simulink model "five_bots_Observer_Obstacle_1_sin_cir"  (R2019b)
settings: Solver=ode5  StartTime=0.0  StopTime=35.0  FixedStep=0.005  RelTol=1e-3
(part 1 of 3)
settings Model: Creator=a1752760  LastModifiedBy=a1752760
settings DataIOCC: ReturnWorkspaceOutputs=off
settings DebuggingCC: ArithmeticOperatorsInVariantConditions=warning
settings SFSimCC: CustomCodeUndefinedFunction=UseInterfaceOnly

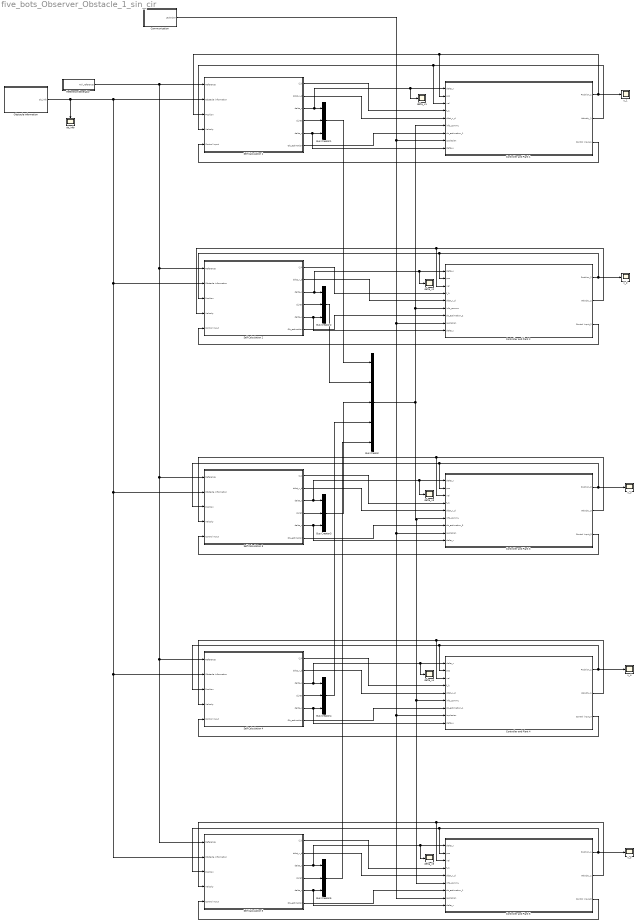
== system five_bots_Observer_Obstacle_1_sin_cir ==
  Bus Creator : BusCreator  Inputs=5
  Bus Creator{1..5} (5 alike) : BusCreator  Inputs=3
  Communication : Subsystem
  Controller and Plant 1 : Subsystem
  Controller and Plant 2 : Subsystem
  Controller and Plant 3 : Subsystem
  Controller and Plant 4 : Subsystem
  Controller and Plant 5 : Subsystem
  Obstacle Information : MATLAB Function  TreatAsAtomicUnit=on
  Reference Generator : Subsystem
  Self Calculation 1 : Subsystem
  Self Calculation 2 : Subsystem
  Self Calculation 3 : Subsystem
  Self Calculation 4 : Subsystem
  Self Calculation 5 : Subsystem
  delta_x{1..5} (5 alike) : Scope
  ob_info : Scope
  x_{1..5} (5 alike) : Scope
  wires:
  Obstacle Information/1(ob_info) -> Self Calculation 5/2(Obstacle information), Self Calculation 4/2(Obstacle information), Self Calculation 3/2(Obstacle information), Self Calculation 2/2(Obstacle information), Self Calculation 1/2(Obstacle information), ob_info/1
  Reference Generator/1(Full_reference) -> Self Calculation 5/1(Reference), Self Calculation 4/1(Reference), Self Calculation 3/1(Reference), Self Calculation 2/1(Reference), Self Calculation 1/1(Reference)
  Controller and Plant 1/1(Position_1) -> Controller and Plant 1/2(pos), Self Calculation 1/3(Position), x_1/1
  Controller and Plant 1/2(Velocity_1) -> Controller and Plant 1/3(vel), Self Calculation 1/4(Velocity)
  Self Calculation 1/1(f_ik) -> Controller and Plant 1/4(f_ik)
  Self Calculation 1/2(ddot_x_d) -> Controller and Plant 1/5(ddot_x_d)
  Self Calculation 1/6(Ob_estimation) -> Controller and Plant 1/7(ob_estimation_1)
  Self Calculation 1/5(delta_v) -> Controller and Plant 1/9(delta_v), Bus Creator1/3
  Self Calculation 1/4(d_hat) -> Bus Creator1/2
  Self Calculation 1/3(delta_x) -> delta_x1/1, Controller and Plant 1/1(delta_x), Bus Creator1/1
  Controller and Plant 1/3(Control input_1) -> Self Calculation 1/5(Control Input)
  Bus Creator1/1 -> Bus Creator/1
  Bus Creator/1 -> Controller and Plant 2/6(info_commu), Controller and Plant 1/6(info_commu), Controller and Plant 5/6(info_commu), Controller and Plant 4/6(info_commu), Controller and Plant 3/6(info_commu)
  Self Calculation 2/1(f_ik) -> Controller and Plant 2/4(f_ik)
  Self Calculation 2/3(delta_x) -> delta_x2/1, Controller and Plant 2/1(delta_x), Bus Creator2/1
  Self Calculation 2/6(Ob_estimation) -> Controller and Plant 2/7(ob_estimation_2)
  Controller and Plant 2/1(Position_2) -> Self Calculation 2/3(Position), Controller and Plant 2/2(pos), x_2/1
  Self Calculation 2/5(delta_v) -> Controller and Plant 2/9(delta_v), Bus Creator2/3
  Controller and Plant 2/2(Velocity_2) -> Controller and Plant 2/3(vel), Self Calculation 2/4(Velocity)
  Self Calculation 2/4(d_hat) -> Bus Creator2/2
  Self Calculation 2/2(ddot_x_d) -> Controller and Plant 2/5(ddot_x_d)
  Controller and Plant 2/3(Control input_2) -> Self Calculation 2/5(Control Input)
  Controller and Plant 3/3(Control input_3) -> Self Calculation 3/5(Control Input)
  Controller and Plant 3/2(Velocity_3) -> Self Calculation 3/4(Velocity), Controller and Plant 3/3(vel)
  Self Calculation 3/1(f_ik) -> Controller and Plant 3/4(f_ik)
  Self Calculation 3/3(delta_x) -> delta_x3/1, Controller and Plant 3/1(delta_x), Bus Creator3/1
  Controller and Plant 3/1(Position_3) -> Self Calculation 3/3(Position), Controller and Plant 3/2(pos), x_3/1
  Self Calculation 3/4(d_hat) -> Bus Creator3/2
  Self Calculation 3/5(delta_v) -> Controller and Plant 3/9(delta_v), Bus Creator3/3
  Self Calculation 3/6(Ob_estimation) -> Controller and Plant 3/7(ob_estimation_3)
  Self Calculation 3/2(ddot_x_d) -> Controller and Plant 3/5(ddot_x_d)
  Controller and Plant 4/3(Control input_4) -> Self Calculation 4/5(Control Input)
  Controller and Plant 4/2(Velocity_1) -> Self Calculation 4/4(Velocity), Controller and Plant 4/3(vel)
  Self Calculation 4/1(f_ik) -> Controller and Plant 4/4(f_ik)
  Self Calculation 4/3(delta_x) -> delta_x4/1, Controller and Plant 4/1(delta_x), Bus Creator4/1
  Controller and Plant 4/1(Position_1) -> Self Calculation 4/3(Position), Controller and Plant 4/2(pos), x_4/1
  Self Calculation 4/4(d_hat) -> Bus Creator4/2
  Self Calculation 4/5(delta_v) -> Controller and Plant 4/9(delta_v), Bus Creator4/3
  Self Calculation 4/6(Ob_estimation) -> Controller and Plant 4/7(ob_estimation_1)
  Self Calculation 4/2(ddot_x_d) -> Controller and Plant 4/5(ddot_x_d)
  Controller and Plant 5/3(Control input_5) -> Self Calculation 5/5(Control Input)
  Controller and Plant 5/2(Velocity_1) -> Self Calculation 5/4(Velocity), Controller and Plant 5/3(vel)
  Self Calculation 5/1(f_ik) -> Controller and Plant 5/4(f_ik)
  Self Calculation 5/3(delta_x) -> delta_x5/1, Controller and Plant 5/1(delta_x), Bus Creator5/1
  Controller and Plant 5/1(Position_1) -> Self Calculation 5/3(Position), Controller and Plant 5/2(pos), x_5/1
  Self Calculation 5/4(d_hat) -> Bus Creator5/2
  Self Calculation 5/5(delta_v) -> Controller and Plant 5/9(delta_v), Bus Creator5/3
  Communication/1(Laplacian) -> Controller and Plant 5/8(Laplacian), Controller and Plant 4/8(Laplacian), Controller and Plant 3/8(Laplacian), Controller and Plant 2/8(Laplacian), Controller and Plant 1/8(Laplacian)
  Self Calculation 5/6(Ob_estimation) -> Controller and Plant 5/7(ob_estimation_1)
  Self Calculation 5/2(ddot_x_d) -> Controller and Plant 5/5(ddot_x_d)
  Bus Creator2/1 -> Bus Creator/2
  Bus Creator3/1 -> Bus Creator/3
  Bus Creator4/1 -> Bus Creator/4
  Bus Creator5/1 -> Bus Creator/5

== system five_bots_Observer_Obstacle_1_sin_cir/Communication ==
  Add : Sum
  Communication Topology : Constant  Value=[2,0,0,-1,-1;-1,3,-1,-1,0;0,0,1,-1,0;-1,0,0,1,0;0,-1,0,-1,2]  VectorParams1D=off
  Constant : Constant  Value=2  VectorParams1D=off
  Product : Product
  Reference Feeding : Constant  Value=[1,0,0,0,0;0,1,0,0,0;0,0,1,0,0;0,0,0,1,0;0,0,0,0,1]  VectorParams1D=off
  Laplacian : Outport  VectorParamsAs1DForOutWhenUnconnected=off
  wires:
  Constant/1 -> Product/2
  Reference Feeding/1 -> Product/1
  Communication Topology/1 -> Add/1
  Product/1 -> Add/2
  Add/1 -> Laplacian/1

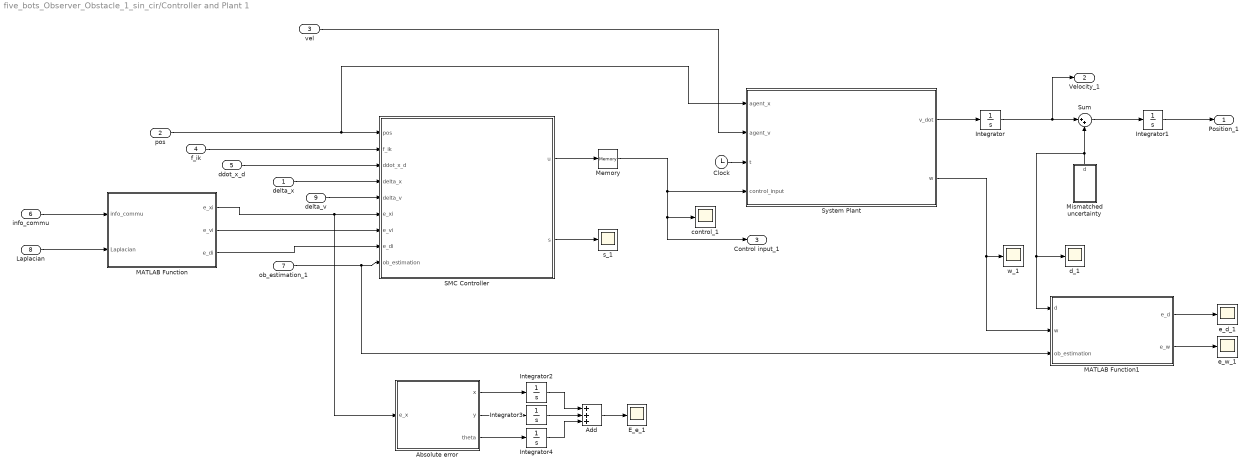
== system five_bots_Observer_Obstacle_1_sin_cir/Controller and Plant 1 ==
  delta_x : Inport
  pos : Inport  Port=2
  vel : Inport  Port=3
  f_ik : Inport  Port=4
  ddot_x_d : Inport  Port=5
  info_commu : Inport  Port=6
  ob_estimation_1 : Inport  Port=7
  Laplacian : Inport  Port=8
  delta_v : Inport  Port=9
  Absolute error : MATLAB Function  TreatAsAtomicUnit=on
  Add : Sum  Inputs=+++
  Clock : Clock
  E_e_1 : Scope
  Integrator : Integrator  InitialCondition=[0;0;0]  ContinuousStateAttributes='speed'
  Integrator1 : Integrator  Tag=Position_x1  InitialCondition=[-0;0.8;pi/6]  ContinuousStateAttributes='position'
  Integrator2 : Integrator  ContinuousStateAttributes='speed'
  Integrator3 : Integrator  ContinuousStateAttributes='speed'
  Integrator4 : Integrator  ContinuousStateAttributes='speed'
  MATLAB Function : MATLAB Function  TreatAsAtomicUnit=on
  MATLAB Function1 : MATLAB Function  TreatAsAtomicUnit=on
  Memory : Memory  InitialCondition=[0;0;0]
  Mismatched uncertainty : Subsystem
  SMC Controller : MATLAB Function  TreatAsAtomicUnit=on
  Sum : Sum  Inputs=|++
  System Plant : MATLAB Function  TreatAsAtomicUnit=on
  control_1 : Scope
  d_1 : Scope
  e_d_1 : Scope
  e_w_1 : Scope
  s_1 : Scope
  w_1 : Scope
  Position_1 : Outport
  Velocity_1 : Outport  Port=2
  Control input_1 : Outport  Port=3
  wires:
  MATLAB Function1/1(e_d) -> e_d_1/1
  Mismatched uncertainty/1(d) -> d_1/1, MATLAB Function1/1(d), Sum/2
  System Plant/1(v_dot) -> Integrator/1
  System Plant/2(w) -> MATLAB Function1/2(w), w_1/1
  Sum/1 -> Integrator1/1
  SMC Controller/2(s) -> s_1/1
  ob_estimation_1/1 -> MATLAB Function1/3(ob_estimation), SMC Controller/9(ob_estimation)
  Integrator1/1 -> Position_1/1
  Clock/1 -> System Plant/3(t)
  Integrator/1 -> Velocity_1/1, Sum/1
  Memory/1 -> System Plant/4(control_input), Control input_1/1, control_1/1
  SMC Controller/1(u) -> Memory/1
  MATLAB Function1/2(e_w) -> e_w_1/1
  pos/1 -> System Plant/1(agent_x), SMC Controller/1(pos)
  vel/1 -> System Plant/2(agent_v)
  f_ik/1 -> SMC Controller/2(f_ik)
  ddot_x_d/1 -> SMC Controller/3(ddot_x_d)
  MATLAB Function/1(e_xi) -> SMC Controller/6(e_xi), Absolute error/1(e_x)
  MATLAB Function/2(e_vi) -> SMC Controller/7(e_vi)
  MATLAB Function/3(e_di) -> SMC Controller/8(e_di)
  info_commu/1 -> MATLAB Function/1(info_commu)
  Laplacian/1 -> MATLAB Function/2(Laplacian)
  Absolute error/2(y) -> Integrator3/1
  Integrator3/1 -> Add/2
  Absolute error/1(x) -> Integrator2/1
  Integrator2/1 -> Add/1
  Integrator4/1 -> Add/3
  Absolute error/3(theta) -> Integrator4/1
  Add/1 -> E_e_1/1
  delta_x/1 -> SMC Controller/4(delta_x)
  delta_v/1 -> SMC Controller/5(delta_v)

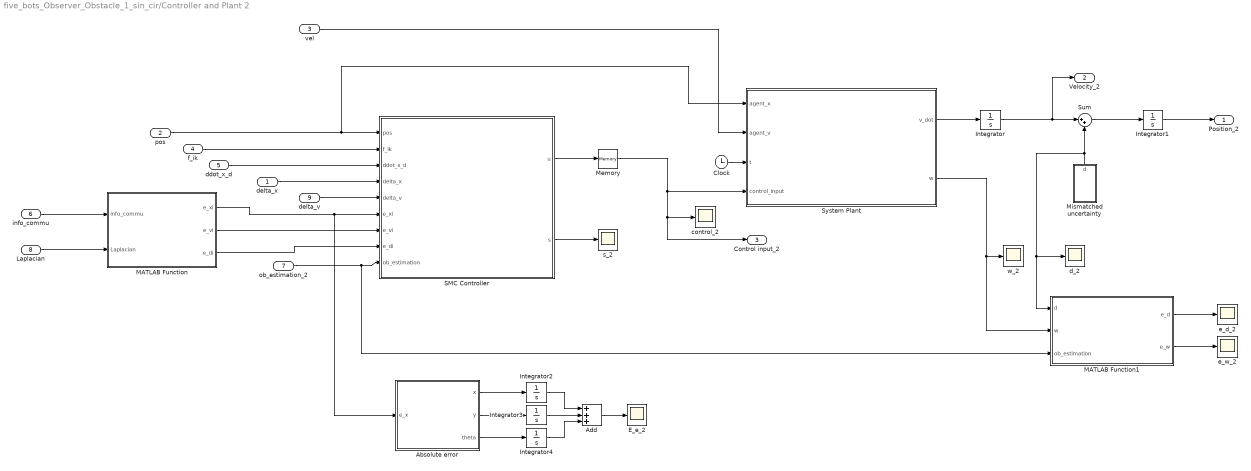
== system five_bots_Observer_Obstacle_1_sin_cir/Controller and Plant 2 ==
  delta_x : Inport
  pos : Inport  Port=2
  vel : Inport  Port=3
  f_ik : Inport  Port=4
  ddot_x_d : Inport  Port=5
  info_commu : Inport  Port=6
  ob_estimation_2 : Inport  Port=7
  Laplacian : Inport  Port=8
  delta_v : Inport  Port=9
  Absolute error : MATLAB Function  TreatAsAtomicUnit=on
  Add : Sum  Inputs=+++
  Clock : Clock
  E_e_2 : Scope
  Integrator : Integrator  InitialCondition=[0;0;0]  ContinuousStateAttributes='speed'
  Integrator1 : Integrator  Tag=Position_x1  InitialCondition=[-1.3;1.4;pi/3]  ContinuousStateAttributes='position'
  Integrator2 : Integrator  ContinuousStateAttributes='speed'
  Integrator3 : Integrator  ContinuousStateAttributes='speed'
  Integrator4 : Integrator  ContinuousStateAttributes='speed'
  MATLAB Function : MATLAB Function  TreatAsAtomicUnit=on
  MATLAB Function1 : MATLAB Function  TreatAsAtomicUnit=on
  Memory : Memory  InitialCondition=[0;0;0]
  Mismatched uncertainty : Subsystem
  SMC Controller : MATLAB Function  TreatAsAtomicUnit=on
  Sum : Sum  Inputs=|++
  System Plant : MATLAB Function  TreatAsAtomicUnit=on
  control_2 : Scope
  d_2 : Scope
  e_d_2 : Scope
  e_w_2 : Scope
  s_2 : Scope
  w_2 : Scope
  Position_2 : Outport
  Velocity_2 : Outport  Port=2
  Control input_2 : Outport  Port=3
  wires:
  MATLAB Function1/1(e_d) -> e_d_2/1
  Mismatched uncertainty/1(d) -> d_2/1, MATLAB Function1/1(d), Sum/2
  System Plant/1(v_dot) -> Integrator/1
  System Plant/2(w) -> MATLAB Function1/2(w), w_2/1
  Sum/1 -> Integrator1/1
  SMC Controller/2(s) -> s_2/1
  ob_estimation_2/1 -> MATLAB Function1/3(ob_estimation), SMC Controller/9(ob_estimation)
  Integrator1/1 -> Position_2/1
  Clock/1 -> System Plant/3(t)
  Integrator/1 -> Velocity_2/1, Sum/1
  Memory/1 -> System Plant/4(control_input), Control input_2/1, control_2/1
  SMC Controller/1(u) -> Memory/1
  MATLAB Function1/2(e_w) -> e_w_2/1
  pos/1 -> System Plant/1(agent_x), SMC Controller/1(pos)
  vel/1 -> System Plant/2(agent_v)
  f_ik/1 -> SMC Controller/2(f_ik)
  ddot_x_d/1 -> SMC Controller/3(ddot_x_d)
  MATLAB Function/1(e_xi) -> SMC Controller/6(e_xi), Absolute error/1(e_x)
  MATLAB Function/2(e_vi) -> SMC Controller/7(e_vi)
  MATLAB Function/3(e_di) -> SMC Controller/8(e_di)
  info_commu/1 -> MATLAB Function/1(info_commu)
  Laplacian/1 -> MATLAB Function/2(Laplacian)
  Absolute error/2(y) -> Integrator3/1
  Integrator3/1 -> Add/2
  Absolute error/1(x) -> Integrator2/1
  Integrator2/1 -> Add/1
  Integrator4/1 -> Add/3
  Absolute error/3(theta) -> Integrator4/1
  Add/1 -> E_e_2/1
  delta_x/1 -> SMC Controller/4(delta_x)
  delta_v/1 -> SMC Controller/5(delta_v)

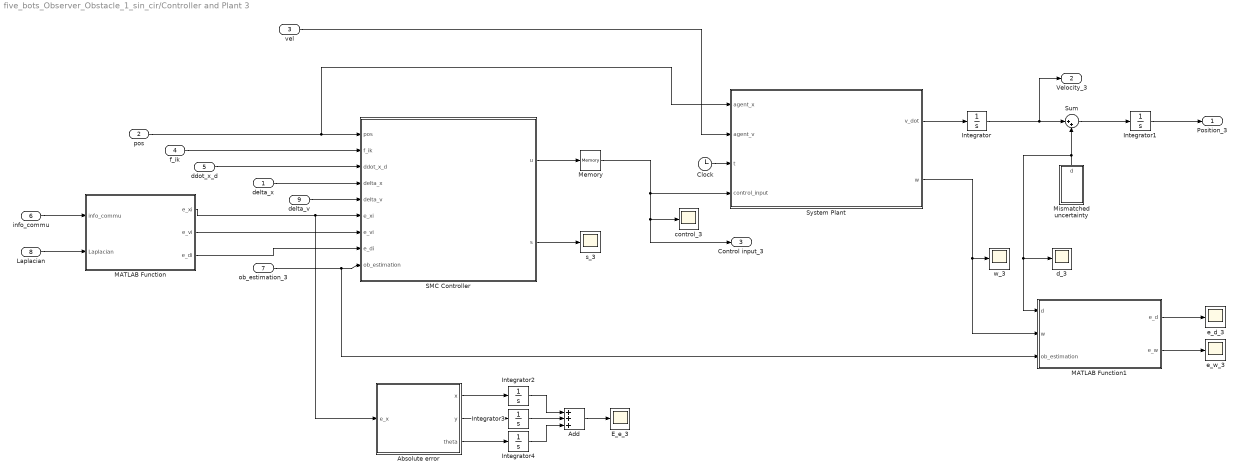
== system five_bots_Observer_Obstacle_1_sin_cir/Controller and Plant 3 ==
  delta_x : Inport
  pos : Inport  Port=2
  vel : Inport  Port=3
  f_ik : Inport  Port=4
  ddot_x_d : Inport  Port=5
  info_commu : Inport  Port=6
  ob_estimation_3 : Inport  Port=7
  Laplacian : Inport  Port=8
  delta_v : Inport  Port=9
  Absolute error : MATLAB Function  TreatAsAtomicUnit=on
  Add : Sum  Inputs=+++
  Clock : Clock
  E_e_3 : Scope
  Integrator : Integrator  InitialCondition=[0;0;0]  ContinuousStateAttributes='speed'
  Integrator1 : Integrator  Tag=Position_x1  InitialCondition=[-1.4;-1.2;-pi/4]  ContinuousStateAttributes='position'
  Integrator2 : Integrator  ContinuousStateAttributes='speed'
  Integrator3 : Integrator  ContinuousStateAttributes='speed'
  Integrator4 : Integrator  ContinuousStateAttributes='speed'
  MATLAB Function : MATLAB Function  TreatAsAtomicUnit=on
  MATLAB Function1 : MATLAB Function  TreatAsAtomicUnit=on
  Memory : Memory  InitialCondition=[0;0;0]
  Mismatched uncertainty : Subsystem
  SMC Controller : MATLAB Function  TreatAsAtomicUnit=on
  Sum : Sum  Inputs=|++
  System Plant : MATLAB Function  TreatAsAtomicUnit=on
  control_3 : Scope
  d_3 : Scope
  e_d_3 : Scope
  e_w_3 : Scope
  s_3 : Scope
  w_3 : Scope
  Position_3 : Outport
  Velocity_3 : Outport  Port=2
  Control input_3 : Outport  Port=3
  wires:
  MATLAB Function1/1(e_d) -> e_d_3/1
  Mismatched uncertainty/1(d) -> d_3/1, MATLAB Function1/1(d), Sum/2
  System Plant/1(v_dot) -> Integrator/1
  System Plant/2(w) -> MATLAB Function1/2(w), w_3/1
  Sum/1 -> Integrator1/1
  SMC Controller/2(s) -> s_3/1
  ob_estimation_3/1 -> MATLAB Function1/3(ob_estimation), SMC Controller/9(ob_estimation)
  Integrator1/1 -> Position_3/1
  Clock/1 -> System Plant/3(t)
  Integrator/1 -> Velocity_3/1, Sum/1
  Memory/1 -> System Plant/4(control_input), Control input_3/1, control_3/1
  SMC Controller/1(u) -> Memory/1
  MATLAB Function1/2(e_w) -> e_w_3/1
  pos/1 -> System Plant/1(agent_x), SMC Controller/1(pos)
  vel/1 -> System Plant/2(agent_v)
  f_ik/1 -> SMC Controller/2(f_ik)
  ddot_x_d/1 -> SMC Controller/3(ddot_x_d)
  MATLAB Function/1(e_xi) -> SMC Controller/6(e_xi), Absolute error/1(e_x)
  MATLAB Function/2(e_vi) -> SMC Controller/7(e_vi)
  MATLAB Function/3(e_di) -> SMC Controller/8(e_di)
  info_commu/1 -> MATLAB Function/1(info_commu)
  Laplacian/1 -> MATLAB Function/2(Laplacian)
  Absolute error/2(y) -> Integrator3/1
  Integrator3/1 -> Add/2
  Absolute error/1(x) -> Integrator2/1
  Integrator2/1 -> Add/1
  Integrator4/1 -> Add/3
  Absolute error/3(theta) -> Integrator4/1
  Add/1 -> E_e_3/1
  delta_x/1 -> SMC Controller/4(delta_x)
  delta_v/1 -> SMC Controller/5(delta_v)

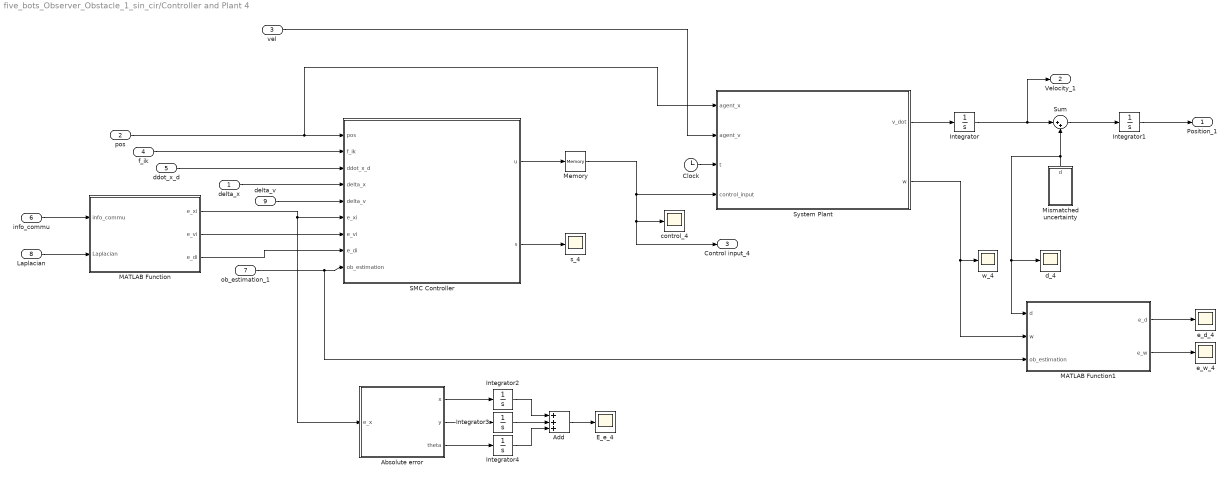
== system five_bots_Observer_Obstacle_1_sin_cir/Controller and Plant 4 ==
  delta_x : Inport
  pos : Inport  Port=2
  vel : Inport  Port=3
  f_ik : Inport  Port=4
  ddot_x_d : Inport  Port=5
  info_commu : Inport  Port=6
  ob_estimation_1 : Inport  Port=7
  Laplacian : Inport  Port=8
  delta_v : Inport  Port=9
  Absolute error : MATLAB Function  TreatAsAtomicUnit=on
  Add : Sum  Inputs=+++
  Clock : Clock
  E_e_4 : Scope
  Integrator : Integrator  InitialCondition=[0;0;0]  ContinuousStateAttributes='speed'
  Integrator1 : Integrator  Tag=Position_x1  InitialCondition=[0;-0.6;-pi/6]  ContinuousStateAttributes='position'
  Integrator2 : Integrator  ContinuousStateAttributes='speed'
  Integrator3 : Integrator  ContinuousStateAttributes='speed'
  Integrator4 : Integrator  ContinuousStateAttributes='speed'
  MATLAB Function : MATLAB Function  TreatAsAtomicUnit=on
  MATLAB Function1 : MATLAB Function  TreatAsAtomicUnit=on
  Memory : Memory  InitialCondition=[0;0;0]
  Mismatched uncertainty : Subsystem
  SMC Controller : MATLAB Function  TreatAsAtomicUnit=on
  Sum : Sum  Inputs=|++
  System Plant : MATLAB Function  TreatAsAtomicUnit=on
  control_4 : Scope
  d_4 : Scope
  e_d_4 : Scope
  e_w_4 : Scope
  s_4 : Scope
  w_4 : Scope
  Position_1 : Outport
  Velocity_1 : Outport  Port=2
  Control input_4 : Outport  Port=3
  wires:
  MATLAB Function1/1(e_d) -> e_d_4/1
  Mismatched uncertainty/1(d) -> d_4/1, MATLAB Function1/1(d), Sum/2
  System Plant/1(v_dot) -> Integrator/1
  System Plant/2(w) -> MATLAB Function1/2(w), w_4/1
  Sum/1 -> Integrator1/1
  SMC Controller/2(s) -> s_4/1
  ob_estimation_1/1 -> MATLAB Function1/3(ob_estimation), SMC Controller/9(ob_estimation)
  Integrator1/1 -> Position_1/1
  Clock/1 -> System Plant/3(t)
  Integrator/1 -> Velocity_1/1, Sum/1
  Memory/1 -> System Plant/4(control_input), Control input_4/1, control_4/1
  SMC Controller/1(u) -> Memory/1
  MATLAB Function1/2(e_w) -> e_w_4/1
  pos/1 -> System Plant/1(agent_x), SMC Controller/1(pos)
  vel/1 -> System Plant/2(agent_v)
  f_ik/1 -> SMC Controller/2(f_ik)
  ddot_x_d/1 -> SMC Controller/3(ddot_x_d)
  MATLAB Function/1(e_xi) -> SMC Controller/6(e_xi), Absolute error/1(e_x)
  MATLAB Function/2(e_vi) -> SMC Controller/7(e_vi)
  MATLAB Function/3(e_di) -> SMC Controller/8(e_di)
  info_commu/1 -> MATLAB Function/1(info_commu)
  Laplacian/1 -> MATLAB Function/2(Laplacian)
  Absolute error/2(y) -> Integrator3/1
  Integrator3/1 -> Add/2
  Absolute error/1(x) -> Integrator2/1
  Integrator2/1 -> Add/1
  Integrator4/1 -> Add/3
  Absolute error/3(theta) -> Integrator4/1
  Add/1 -> E_e_4/1
  delta_x/1 -> SMC Controller/4(delta_x)
  delta_v/1 -> SMC Controller/5(delta_v)

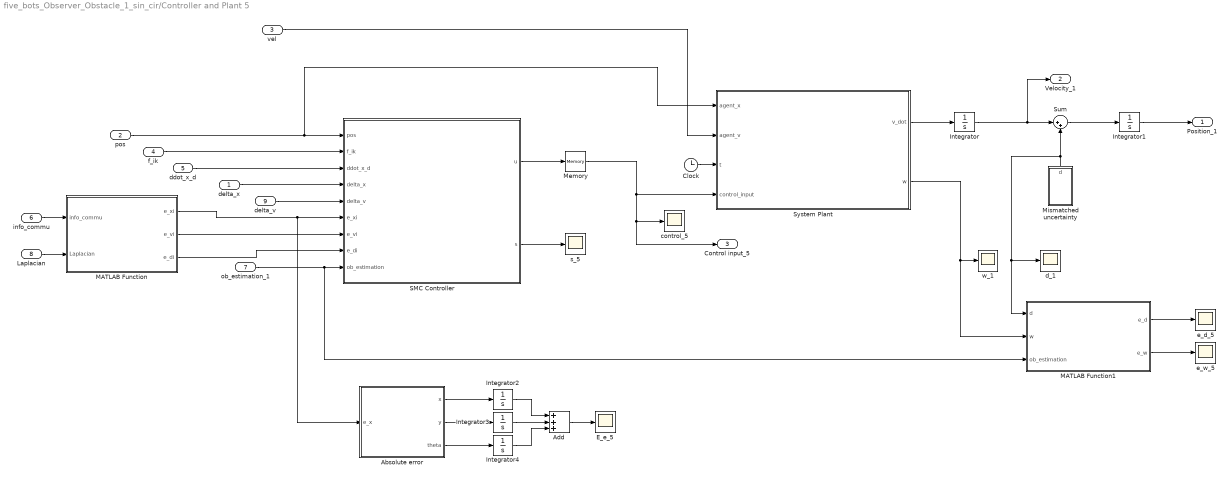
== system five_bots_Observer_Obstacle_1_sin_cir/Controller and Plant 5 ==
  delta_x : Inport
  pos : Inport  Port=2
  vel : Inport  Port=3
  f_ik : Inport  Port=4
  ddot_x_d : Inport  Port=5
  info_commu : Inport  Port=6
  ob_estimation_1 : Inport  Port=7
  Laplacian : Inport  Port=8
  delta_v : Inport  Port=9
  Absolute error : MATLAB Function  TreatAsAtomicUnit=on
  Add : Sum  Inputs=+++
  Clock : Clock
  E_e_5 : Scope
  Integrator : Integrator  InitialCondition=[0;0;0]  ContinuousStateAttributes='speed'
  Integrator1 : Integrator  Tag=Position_x1  InitialCondition=[0.8;0.3;pi/4]  ContinuousStateAttributes='position'
  Integrator2 : Integrator  ContinuousStateAttributes='speed'
  Integrator3 : Integrator  ContinuousStateAttributes='speed'
  Integrator4 : Integrator  ContinuousStateAttributes='speed'
  MATLAB Function : MATLAB Function  TreatAsAtomicUnit=on
  MATLAB Function1 : MATLAB Function  TreatAsAtomicUnit=on
  Memory : Memory  InitialCondition=[0;0;0]
  Mismatched uncertainty : Subsystem
  SMC Controller : MATLAB Function  TreatAsAtomicUnit=on
  Sum : Sum  Inputs=|++
  System Plant : MATLAB Function  TreatAsAtomicUnit=on
  control_5 : Scope
  d_1 : Scope
  e_d_5 : Scope
  e_w_5 : Scope
  s_5 : Scope
  w_1 : Scope
  Position_1 : Outport
  Velocity_1 : Outport  Port=2
  Control input_5 : Outport  Port=3
  wires:
  MATLAB Function1/1(e_d) -> e_d_5/1
  Mismatched uncertainty/1(d) -> d_1/1, MATLAB Function1/1(d), Sum/2
  System Plant/1(v_dot) -> Integrator/1
  System Plant/2(w) -> MATLAB Function1/2(w), w_1/1
  Sum/1 -> Integrator1/1
  SMC Controller/2(s) -> s_5/1
  ob_estimation_1/1 -> MATLAB Function1/3(ob_estimation), SMC Controller/9(ob_estimation)
  Integrator1/1 -> Position_1/1
  Clock/1 -> System Plant/3(t)
  Integrator/1 -> Velocity_1/1, Sum/1
  Memory/1 -> System Plant/4(control_input), Control input_5/1, control_5/1
  SMC Controller/1(u) -> Memory/1
  MATLAB Function1/2(e_w) -> e_w_5/1
  pos/1 -> System Plant/1(agent_x), SMC Controller/1(pos)
  vel/1 -> System Plant/2(agent_v)
  f_ik/1 -> SMC Controller/2(f_ik)
  ddot_x_d/1 -> SMC Controller/3(ddot_x_d)
  MATLAB Function/1(e_xi) -> Absolute error/1(e_x), SMC Controller/6(e_xi)
  MATLAB Function/2(e_vi) -> SMC Controller/7(e_vi)
  MATLAB Function/3(e_di) -> SMC Controller/8(e_di)
  info_commu/1 -> MATLAB Function/1(info_commu)
  Laplacian/1 -> MATLAB Function/2(Laplacian)
  Absolute error/2(y) -> Integrator3/1
  Integrator3/1 -> Add/2
  Absolute error/1(x) -> Integrator2/1
  Integrator2/1 -> Add/1
  Integrator4/1 -> Add/3
  Absolute error/3(theta) -> Integrator4/1
  Add/1 -> E_e_5/1
  delta_x/1 -> SMC Controller/4(delta_x)
  delta_v/1 -> SMC Controller/5(delta_v)

== system five_bots_Observer_Obstacle_1_sin_cir/Reference Generator ==
  Acceleration reference : MATLAB Function  TreatAsAtomicUnit=on
  Acceleration_ref : Scope
  Bus Creator1 : BusCreator  Inputs=3
  Clock : Clock
  Position Reference : MATLAB Function  TreatAsAtomicUnit=on
  Position_ref : Scope
  Speed Reference : MATLAB Function  TreatAsAtomicUnit=on
  Speed_ref : Scope
  Full_reference : Outport  VectorParamsAs1DForOutWhenUnconnected=off
  wires:
  Clock/1 -> Position Reference/1(t), Acceleration reference/1(t), Speed Reference/1(t)
  Position Reference/1(x1d) -> Position_ref/1, Bus Creator1/1
  Speed Reference/1(x2d) -> Speed_ref/1, Bus Creator1/2
  Acceleration reference/1(x2d_dot) -> Acceleration_ref/1, Bus Creator1/3
  Bus Creator1/1 -> Full_reference/1

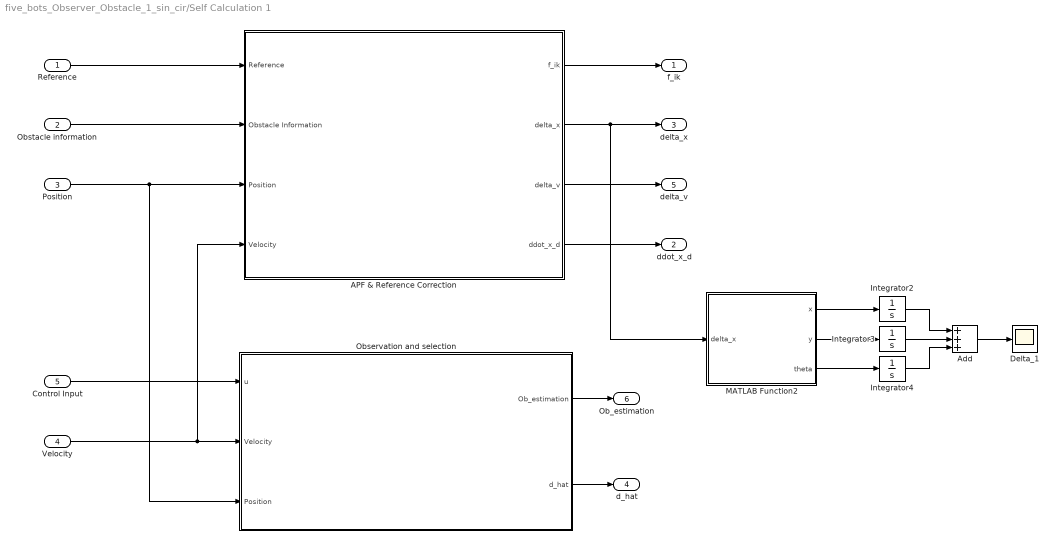
== system five_bots_Observer_Obstacle_1_sin_cir/Self Calculation 1 ==
  Reference : Inport
  Obstacle information : Inport  Port=2
  Position : Inport  Port=3
  Velocity : Inport  Port=4
  Control Input : Inport  Port=5
  APF & Reference Correction : Subsystem
  Add : Sum  Inputs=+++
  Delta_1 : Scope
  Integrator2 : Integrator  ContinuousStateAttributes='speed'
  Integrator3 : Integrator  ContinuousStateAttributes='speed'
  Integrator4 : Integrator  ContinuousStateAttributes='speed'
  MATLAB Function2 : MATLAB Function  TreatAsAtomicUnit=on
  Observation and selection : Subsystem
  f_ik : Outport
  ddot_x_d : Outport  Port=2
  delta_x : Outport  Port=3
  d_hat : Outport  Port=4
  delta_v : Outport  Port=5
  Ob_estimation : Outport  Port=6
  wires:
  Position/1 -> Observation and selection/3(Position), APF & Reference Correction/3(Position)
  Obstacle information/1 -> APF & Reference Correction/2(Obstacle Information)
  Reference/1 -> APF & Reference Correction/1(Reference)
  Velocity/1 -> APF & Reference Correction/4(Velocity), Observation and selection/2(Velocity)
  Control Input/1 -> Observation and selection/1(u)
  Observation and selection/1(Ob_estimation) -> Ob_estimation/1
  Observation and selection/2(d_hat) -> d_hat/1
  APF & Reference Correction/4(ddot_x_d) -> ddot_x_d/1
  APF & Reference Correction/3(delta_v) -> delta_v/1
  APF & Reference Correction/2(delta_x) -> MATLAB Function2/1(delta_x), delta_x/1
  APF & Reference Correction/1(f_ik) -> f_ik/1
  MATLAB Function2/2(y) -> Integrator3/1
  Integrator3/1 -> Add/2
  MATLAB Function2/1(x) -> Integrator2/1
  Integrator2/1 -> Add/1
  Integrator4/1 -> Add/3
  MATLAB Function2/3(theta) -> Integrator4/1
  Add/1 -> Delta_1/1

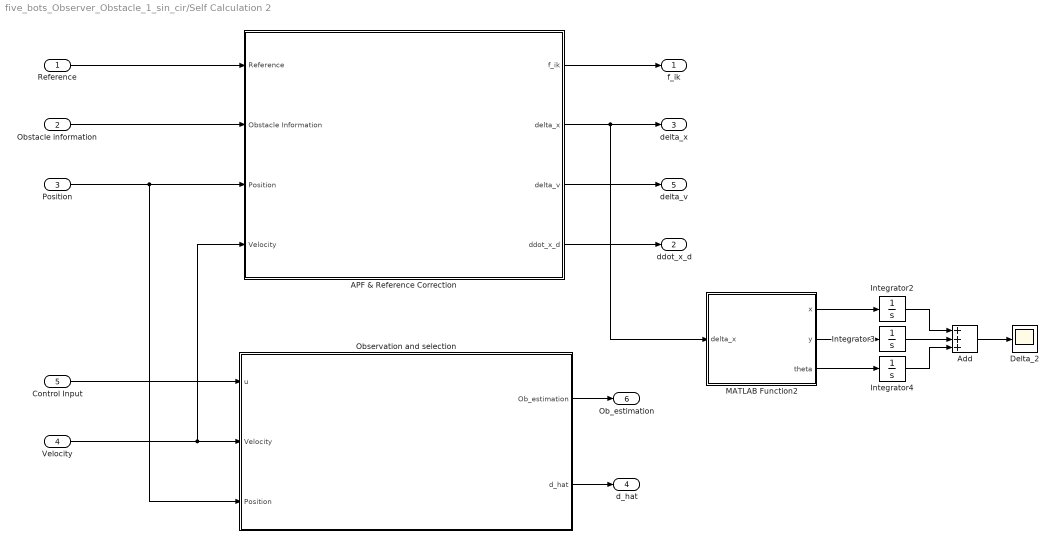
== system five_bots_Observer_Obstacle_1_sin_cir/Self Calculation 2 ==
  Reference : Inport
  Obstacle information : Inport  Port=2
  Position : Inport  Port=3
  Velocity : Inport  Port=4
  Control Input : Inport  Port=5
  APF & Reference Correction : Subsystem
  Add : Sum  Inputs=+++
  Delta_2 : Scope
  Integrator2 : Integrator  ContinuousStateAttributes='speed'
  Integrator3 : Integrator  ContinuousStateAttributes='speed'
  Integrator4 : Integrator  ContinuousStateAttributes='speed'
  MATLAB Function2 : MATLAB Function  TreatAsAtomicUnit=on
  Observation and selection : Subsystem
  f_ik : Outport
  ddot_x_d : Outport  Port=2
  delta_x : Outport  Port=3
  d_hat : Outport  Port=4
  delta_v : Outport  Port=5
  Ob_estimation : Outport  Port=6
  wires:
  Position/1 -> Observation and selection/3(Position), APF & Reference Correction/3(Position)
  Obstacle information/1 -> APF & Reference Correction/2(Obstacle Information)
  Reference/1 -> APF & Reference Correction/1(Reference)
  Velocity/1 -> APF & Reference Correction/4(Velocity), Observation and selection/2(Velocity)
  Control Input/1 -> Observation and selection/1(u)
  Observation and selection/1(Ob_estimation) -> Ob_estimation/1
  Observation and selection/2(d_hat) -> d_hat/1
  APF & Reference Correction/4(ddot_x_d) -> ddot_x_d/1
  APF & Reference Correction/3(delta_v) -> delta_v/1
  APF & Reference Correction/2(delta_x) -> MATLAB Function2/1(delta_x), delta_x/1
  APF & Reference Correction/1(f_ik) -> f_ik/1
  MATLAB Function2/2(y) -> Integrator3/1
  Integrator3/1 -> Add/2
  MATLAB Function2/1(x) -> Integrator2/1
  Integrator2/1 -> Add/1
  Integrator4/1 -> Add/3
  MATLAB Function2/3(theta) -> Integrator4/1
  Add/1 -> Delta_2/1

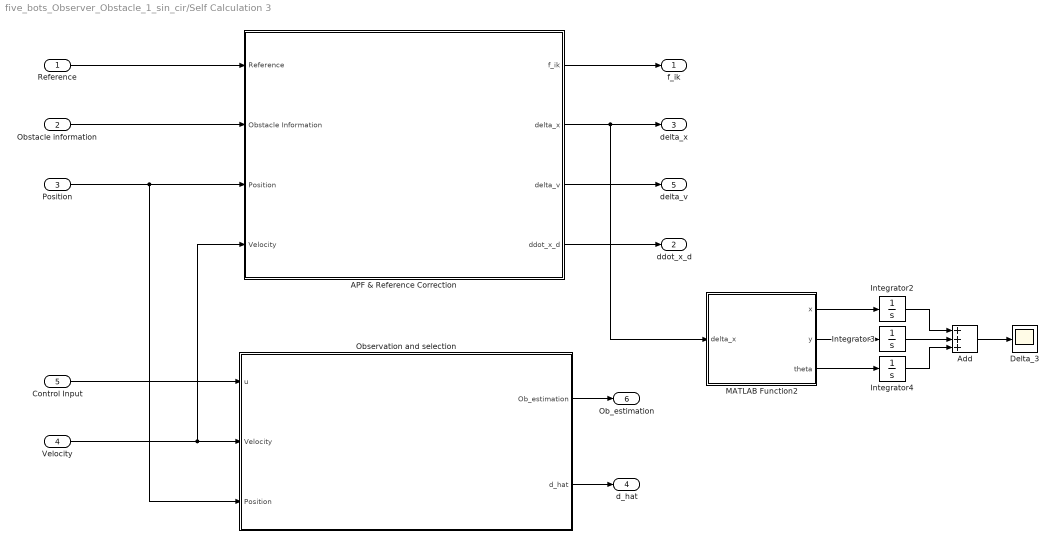
== system five_bots_Observer_Obstacle_1_sin_cir/Self Calculation 3 ==
  Reference : Inport
  Obstacle information : Inport  Port=2
  Position : Inport  Port=3
  Velocity : Inport  Port=4
  Control Input : Inport  Port=5
  APF & Reference Correction : Subsystem
  Add : Sum  Inputs=+++
  Delta_3 : Scope
  Integrator2 : Integrator  ContinuousStateAttributes='speed'
  Integrator3 : Integrator  ContinuousStateAttributes='speed'
  Integrator4 : Integrator  ContinuousStateAttributes='speed'
  MATLAB Function2 : MATLAB Function  TreatAsAtomicUnit=on
  Observation and selection : Subsystem
  f_ik : Outport
  ddot_x_d : Outport  Port=2
  delta_x : Outport  Port=3
  d_hat : Outport  Port=4
  delta_v : Outport  Port=5
  Ob_estimation : Outport  Port=6
  wires:
  Position/1 -> Observation and selection/3(Position), APF & Reference Correction/3(Position)
  Obstacle information/1 -> APF & Reference Correction/2(Obstacle Information)
  Reference/1 -> APF & Reference Correction/1(Reference)
  Velocity/1 -> APF & Reference Correction/4(Velocity), Observation and selection/2(Velocity)
  Control Input/1 -> Observation and selection/1(u)
  Observation and selection/1(Ob_estimation) -> Ob_estimation/1
  Observation and selection/2(d_hat) -> d_hat/1
  APF & Reference Correction/4(ddot_x_d) -> ddot_x_d/1
  APF & Reference Correction/3(delta_v) -> delta_v/1
  APF & Reference Correction/2(delta_x) -> MATLAB Function2/1(delta_x), delta_x/1
  APF & Reference Correction/1(f_ik) -> f_ik/1
  MATLAB Function2/2(y) -> Integrator3/1
  Integrator3/1 -> Add/2
  MATLAB Function2/1(x) -> Integrator2/1
  Integrator2/1 -> Add/1
  Integrator4/1 -> Add/3
  MATLAB Function2/3(theta) -> Integrator4/1
  Add/1 -> Delta_3/1

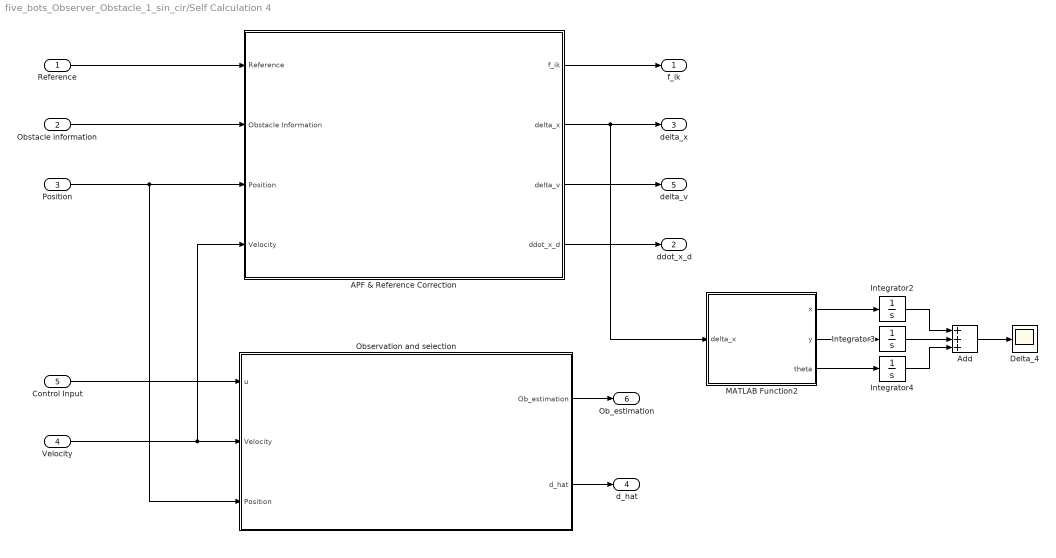
== system five_bots_Observer_Obstacle_1_sin_cir/Self Calculation 4 ==
  Reference : Inport
  Obstacle information : Inport  Port=2
  Position : Inport  Port=3
  Velocity : Inport  Port=4
  Control Input : Inport  Port=5
  APF & Reference Correction : Subsystem
  Add : Sum  Inputs=+++
  Delta_4 : Scope
  Integrator2 : Integrator  ContinuousStateAttributes='speed'
  Integrator3 : Integrator  ContinuousStateAttributes='speed'
  Integrator4 : Integrator  ContinuousStateAttributes='speed'
  MATLAB Function2 : MATLAB Function  TreatAsAtomicUnit=on
  Observation and selection : Subsystem
  f_ik : Outport
  ddot_x_d : Outport  Port=2
  delta_x : Outport  Port=3
  d_hat : Outport  Port=4
  delta_v : Outport  Port=5
  Ob_estimation : Outport  Port=6
  wires:
  Position/1 -> Observation and selection/3(Position), APF & Reference Correction/3(Position)
  Obstacle information/1 -> APF & Reference Correction/2(Obstacle Information)
  Reference/1 -> APF & Reference Correction/1(Reference)
  Velocity/1 -> APF & Reference Correction/4(Velocity), Observation and selection/2(Velocity)
  Control Input/1 -> Observation and selection/1(u)
  Observation and selection/1(Ob_estimation) -> Ob_estimation/1
  Observation and selection/2(d_hat) -> d_hat/1
  APF & Reference Correction/4(ddot_x_d) -> ddot_x_d/1
  APF & Reference Correction/3(delta_v) -> delta_v/1
  APF & Reference Correction/2(delta_x) -> MATLAB Function2/1(delta_x), delta_x/1
  APF & Reference Correction/1(f_ik) -> f_ik/1
  MATLAB Function2/2(y) -> Integrator3/1
  Integrator3/1 -> Add/2
  MATLAB Function2/1(x) -> Integrator2/1
  Integrator2/1 -> Add/1
  Integrator4/1 -> Add/3
  MATLAB Function2/3(theta) -> Integrator4/1
  Add/1 -> Delta_4/1

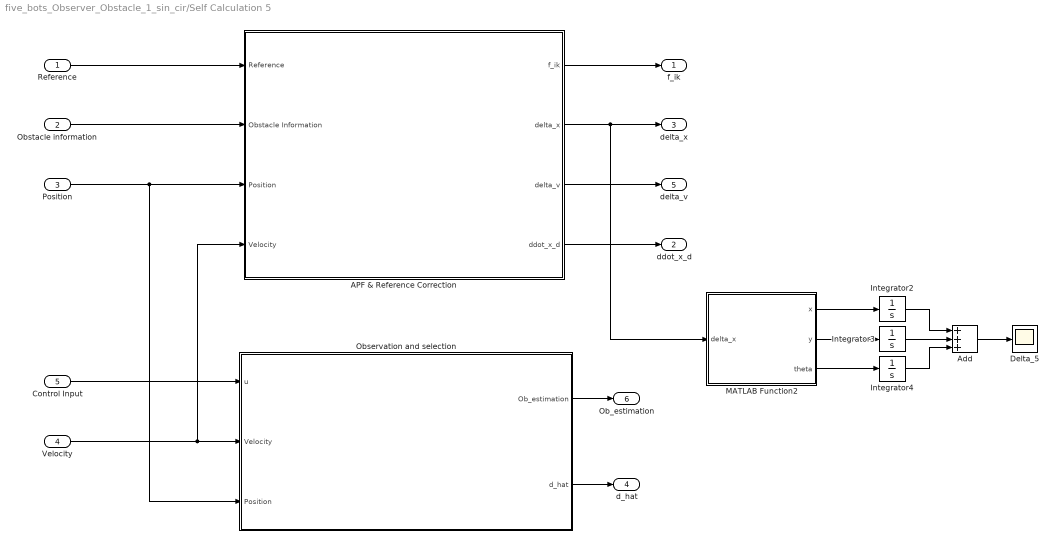
== system five_bots_Observer_Obstacle_1_sin_cir/Self Calculation 5 ==
  Reference : Inport
  Obstacle information : Inport  Port=2
  Position : Inport  Port=3
  Velocity : Inport  Port=4
  Control Input : Inport  Port=5
  APF & Reference Correction : Subsystem
  Add : Sum  Inputs=+++
  Delta_5 : Scope
  Integrator2 : Integrator  ContinuousStateAttributes='speed'
  Integrator3 : Integrator  ContinuousStateAttributes='speed'
  Integrator4 : Integrator  ContinuousStateAttributes='speed'
  MATLAB Function2 : MATLAB Function  TreatAsAtomicUnit=on
  Observation and selection : Subsystem
  f_ik : Outport
  ddot_x_d : Outport  Port=2
  delta_x : Outport  Port=3
  d_hat : Outport  Port=4
  delta_v : Outport  Port=5
  Ob_estimation : Outport  Port=6
  wires:
  Position/1 -> Observation and selection/3(Position), APF & Reference Correction/3(Position)
  Obstacle information/1 -> APF & Reference Correction/2(Obstacle Information)
  Reference/1 -> APF & Reference Correction/1(Reference)
  Velocity/1 -> APF & Reference Correction/4(Velocity), Observation and selection/2(Velocity)
  Control Input/1 -> Observation and selection/1(u)
  Observation and selection/1(Ob_estimation) -> Ob_estimation/1
  Observation and selection/2(d_hat) -> d_hat/1
  APF & Reference Correction/4(ddot_x_d) -> ddot_x_d/1
  APF & Reference Correction/3(delta_v) -> delta_v/1
  APF & Reference Correction/2(delta_x) -> MATLAB Function2/1(delta_x), delta_x/1
  APF & Reference Correction/1(f_ik) -> f_ik/1
  MATLAB Function2/2(y) -> Integrator3/1
  Integrator3/1 -> Add/2
  MATLAB Function2/1(x) -> Integrator2/1
  Integrator2/1 -> Add/1
  Integrator4/1 -> Add/3
  MATLAB Function2/3(theta) -> Integrator4/1
  Add/1 -> Delta_5/1

== system five_bots_Observer_Obstacle_1_sin_cir/Controller and Plant 1/Mismatched uncertainty ==
  Clock1 : Clock
  Mismatched disturbance : MATLAB Function  TreatAsAtomicUnit=on
  d : Outport
  wires:
  Clock1/1 -> Mismatched disturbance/1(t)
  Mismatched disturbance/1(d) -> d/1

== system five_bots_Observer_Obstacle_1_sin_cir/Controller and Plant 2/Mismatched uncertainty ==
  Clock1 : Clock
  Mismatched disturbance : MATLAB Function  TreatAsAtomicUnit=on
  d : Outport
  wires:
  Clock1/1 -> Mismatched disturbance/1(t)
  Mismatched disturbance/1(d) -> d/1

== system five_bots_Observer_Obstacle_1_sin_cir/Controller and Plant 3/Mismatched uncertainty ==
  Clock1 : Clock
  Mismatched disturbance : MATLAB Function  TreatAsAtomicUnit=on
  d : Outport
  wires:
  Clock1/1 -> Mismatched disturbance/1(t)
  Mismatched disturbance/1(d) -> d/1

== system five_bots_Observer_Obstacle_1_sin_cir/Controller and Plant 4/Mismatched uncertainty ==
  Clock1 : Clock
  Mismatched disturbance : MATLAB Function  TreatAsAtomicUnit=on
  d : Outport
  wires:
  Clock1/1 -> Mismatched disturbance/1(t)
  Mismatched disturbance/1(d) -> d/1

== system five_bots_Observer_Obstacle_1_sin_cir/Controller and Plant 5/Mismatched uncertainty ==
  Clock1 : Clock
  Mismatched disturbance : MATLAB Function  TreatAsAtomicUnit=on
  d : Outport
  wires:
  Clock1/1 -> Mismatched disturbance/1(t)
  Mismatched disturbance/1(d) -> d/1

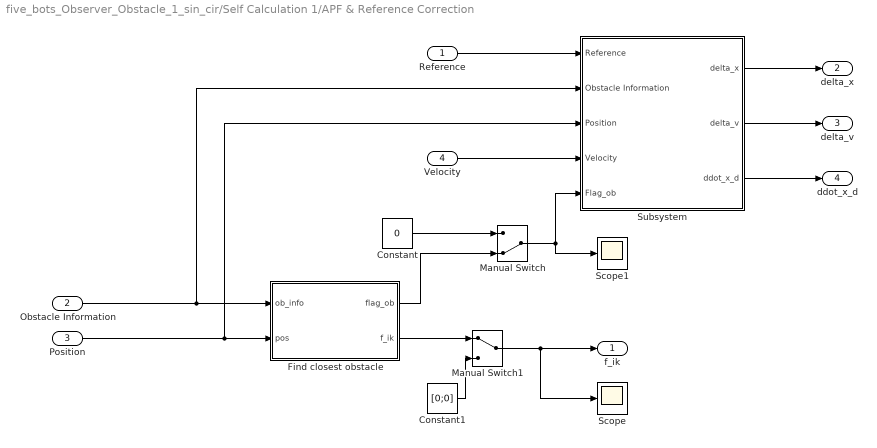
== system five_bots_Observer_Obstacle_1_sin_cir/Self Calculation 1/APF & Reference Correction ==
  Reference : Inport
  Obstacle Information : Inport  Port=2
  Position : Inport  Port=3
  Velocity : Inport  Port=4
  Constant : Constant  Value=0
  Constant1 : Constant  Value=[0;0]
  Find closest obstacle : MATLAB Function  TreatAsAtomicUnit=on
  Manual Switch : ManualSwitch  CurrentSetting=0
  Manual Switch1 : ManualSwitch
  Scope : Scope
  Scope1 : Scope
  Subsystem : Subsystem
  f_ik : Outport
  delta_x : Outport  Port=2
  delta_v : Outport  Port=3
  ddot_x_d : Outport  Port=4
  wires:
  Position/1 -> Subsystem/3(Position), Find closest obstacle/2(pos)
  Obstacle Information/1 -> Subsystem/2(Obstacle Information), Find closest obstacle/1(ob_info)
  Find closest obstacle/1(flag_ob) -> Manual Switch/2
  Constant/1 -> Manual Switch/1
  Manual Switch/1 -> Scope1/1, Subsystem/5(Flag_ob)
  Reference/1 -> Subsystem/1(Reference)
  Subsystem/3(ddot_x_d) -> ddot_x_d/1
  Subsystem/2(delta_v) -> delta_v/1
  Subsystem/1(delta_x) -> delta_x/1
  Velocity/1 -> Subsystem/4(Velocity)
  Find closest obstacle/2(f_ik) -> Manual Switch1/1
  Constant1/1 -> Manual Switch1/2
  Manual Switch1/1 -> Scope/1, f_ik/1

== system five_bots_Observer_Obstacle_1_sin_cir/Self Calculation 1/Observation and selection ==
  u : Inport
  Velocity : Inport  Port=2
  Position : Inport  Port=3
  Control input transfer : MATLAB Function  TreatAsAtomicUnit=on
  Observer : Subsystem
  Scope2 : Scope
  Selecting Information : MATLAB Function  TreatAsAtomicUnit=on
  Ob_estimation : Outport
  d_hat : Outport  Port=2
  wires:
  Selecting Information/1(ob_estimation) -> Ob_estimation/1
  Observer/2(second_hat) -> Selecting Information/2(second_hat)
  Observer/1(first_hat) -> Selecting Information/1(first_hat)
  Observer/3(first_hat_dot) -> Selecting Information/3(first_hat_dot)
  Position/1 -> Control input transfer/2(pos), Observer/3(Position)
  Velocity/1 -> Observer/2(Velocity)
  Control input transfer/1(u_norm) -> Scope2/1, Observer/1(u_norm)
  u/1 -> Control input transfer/1(u)
  Selecting Information/2(d_hat) -> d_hat/1

== system five_bots_Observer_Obstacle_1_sin_cir/Self Calculation 2/APF & Reference Correction ==
  Reference : Inport
  Obstacle Information : Inport  Port=2
  Position : Inport  Port=3
  Velocity : Inport  Port=4
  Constant : Constant  Value=0
  Constant1 : Constant  Value=[0;0]
  Find closest obstacle : MATLAB Function  TreatAsAtomicUnit=on
  Manual Switch : ManualSwitch  CurrentSetting=0
  Manual Switch1 : ManualSwitch
  Scope : Scope
  Scope1 : Scope
  Subsystem : Subsystem
  f_ik : Outport
  delta_x : Outport  Port=2
  delta_v : Outport  Port=3
  ddot_x_d : Outport  Port=4
  wires:
  Position/1 -> Subsystem/3(Position), Find closest obstacle/2(pos)
  Obstacle Information/1 -> Subsystem/2(Obstacle Information), Find closest obstacle/1(ob_info)
  Find closest obstacle/1(flag_ob) -> Manual Switch/2
  Constant/1 -> Manual Switch/1
  Manual Switch/1 -> Scope1/1, Subsystem/5(Flag_ob)
  Reference/1 -> Subsystem/1(Reference)
  Subsystem/3(ddot_x_d) -> ddot_x_d/1
  Subsystem/2(delta_v) -> delta_v/1
  Subsystem/1(delta_x) -> delta_x/1
  Velocity/1 -> Subsystem/4(Velocity)
  Find closest obstacle/2(f_ik) -> Manual Switch1/1
  Constant1/1 -> Manual Switch1/2
  Manual Switch1/1 -> Scope/1, f_ik/1

== system five_bots_Observer_Obstacle_1_sin_cir/Self Calculation 2/Observation and selection ==
  u : Inport
  Velocity : Inport  Port=2
  Position : Inport  Port=3
  Control input transfer : MATLAB Function  TreatAsAtomicUnit=on
  Observer : Subsystem
  Scope2 : Scope
  Selecting Information : MATLAB Function  TreatAsAtomicUnit=on
  Ob_estimation : Outport
  d_hat : Outport  Port=2
  wires:
  Selecting Information/1(ob_estimation) -> Ob_estimation/1
  Observer/2(second_hat) -> Selecting Information/2(second_hat)
  Observer/1(first_hat) -> Selecting Information/1(first_hat)
  Observer/3(first_hat_dot) -> Selecting Information/3(first_hat_dot)
  Position/1 -> Control input transfer/2(pos), Observer/3(Position)
  Velocity/1 -> Observer/2(Velocity)
  Control input transfer/1(u_norm) -> Scope2/1, Observer/1(u_norm)
  u/1 -> Control input transfer/1(u)
  Selecting Information/2(d_hat) -> d_hat/1

== system five_bots_Observer_Obstacle_1_sin_cir/Self Calculation 3/APF & Reference Correction ==
  Reference : Inport
  Obstacle Information : Inport  Port=2
  Position : Inport  Port=3
  Velocity : Inport  Port=4
  Constant : Constant  Value=0
  Constant1 : Constant  Value=[0;0]
  Find closest obstacle : MATLAB Function  TreatAsAtomicUnit=on
  Manual Switch : ManualSwitch  CurrentSetting=0
  Manual Switch1 : ManualSwitch
  Scope : Scope
  Scope1 : Scope
  Subsystem : Subsystem
  f_ik : Outport
  delta_x : Outport  Port=2
  delta_v : Outport  Port=3
  ddot_x_d : Outport  Port=4
  wires:
  Position/1 -> Subsystem/3(Position), Find closest obstacle/2(pos)
  Obstacle Information/1 -> Subsystem/2(Obstacle Information), Find closest obstacle/1(ob_info)
  Find closest obstacle/1(flag_ob) -> Manual Switch/2
  Constant/1 -> Manual Switch/1
  Manual Switch/1 -> Scope1/1, Subsystem/5(Flag_ob)
  Reference/1 -> Subsystem/1(Reference)
  Subsystem/3(ddot_x_d) -> ddot_x_d/1
  Subsystem/2(delta_v) -> delta_v/1
  Subsystem/1(delta_x) -> delta_x/1
  Velocity/1 -> Subsystem/4(Velocity)
  Find closest obstacle/2(f_ik) -> Manual Switch1/1
  Constant1/1 -> Manual Switch1/2
  Manual Switch1/1 -> Scope/1, f_ik/1

== system five_bots_Observer_Obstacle_1_sin_cir/Self Calculation 3/Observation and selection ==
  u : Inport
  Velocity : Inport  Port=2
  Position : Inport  Port=3
  Control input transfer : MATLAB Function  TreatAsAtomicUnit=on
  Observer : Subsystem
  Scope2 : Scope
  Selecting Information : MATLAB Function  TreatAsAtomicUnit=on
  Ob_estimation : Outport
  d_hat : Outport  Port=2
  wires:
  Selecting Information/1(ob_estimation) -> Ob_estimation/1
  Observer/2(second_hat) -> Selecting Information/2(second_hat)
  Observer/1(first_hat) -> Selecting Information/1(first_hat)
  Observer/3(first_hat_dot) -> Selecting Information/3(first_hat_dot)
  Position/1 -> Control input transfer/2(pos), Observer/3(Position)
  Velocity/1 -> Observer/2(Velocity)
  Control input transfer/1(u_norm) -> Scope2/1, Observer/1(u_norm)
  u/1 -> Control input transfer/1(u)
  Selecting Information/2(d_hat) -> d_hat/1

== system five_bots_Observer_Obstacle_1_sin_cir/Self Calculation 4/APF & Reference Correction ==
  Reference : Inport
  Obstacle Information : Inport  Port=2
  Position : Inport  Port=3
  Velocity : Inport  Port=4
  Constant : Constant  Value=0
  Constant1 : Constant  Value=[0;0]
  Find closest obstacle : MATLAB Function  TreatAsAtomicUnit=on
  Manual Switch : ManualSwitch  CurrentSetting=0
  Manual Switch1 : ManualSwitch
  Scope : Scope
  Scope1 : Scope
  Subsystem : Subsystem
  f_ik : Outport
  delta_x : Outport  Port=2
  delta_v : Outport  Port=3
  ddot_x_d : Outport  Port=4
  wires:
  Position/1 -> Subsystem/3(Position), Find closest obstacle/2(pos)
  Obstacle Information/1 -> Subsystem/2(Obstacle Information), Find closest obstacle/1(ob_info)
  Find closest obstacle/1(flag_ob) -> Manual Switch/2
  Constant/1 -> Manual Switch/1
  Manual Switch/1 -> Scope1/1, Subsystem/5(Flag_ob)
  Reference/1 -> Subsystem/1(Reference)
  Subsystem/3(ddot_x_d) -> ddot_x_d/1
  Subsystem/2(delta_v) -> delta_v/1
  Subsystem/1(delta_x) -> delta_x/1
  Velocity/1 -> Subsystem/4(Velocity)
  Find closest obstacle/2(f_ik) -> Manual Switch1/1
  Constant1/1 -> Manual Switch1/2
  Manual Switch1/1 -> Scope/1, f_ik/1

== system five_bots_Observer_Obstacle_1_sin_cir/Self Calculation 4/Observation and selection ==
  u : Inport
  Velocity : Inport  Port=2
  Position : Inport  Port=3
  Control input transfer : MATLAB Function  TreatAsAtomicUnit=on
  Observer : Subsystem
  Scope2 : Scope
  Selecting Information : MATLAB Function  TreatAsAtomicUnit=on
  Ob_estimation : Outport
  d_hat : Outport  Port=2
  wires:
  Selecting Information/1(ob_estimation) -> Ob_estimation/1
  Observer/2(second_hat) -> Selecting Information/2(second_hat)
  Observer/1(first_hat) -> Selecting Information/1(first_hat)
  Observer/3(first_hat_dot) -> Selecting Information/3(first_hat_dot)
  Position/1 -> Control input transfer/2(pos), Observer/3(Position)
  Velocity/1 -> Observer/2(Velocity)
  Control input transfer/1(u_norm) -> Scope2/1, Observer/1(u_norm)
  u/1 -> Control input transfer/1(u)
  Selecting Information/2(d_hat) -> d_hat/1

== system five_bots_Observer_Obstacle_1_sin_cir/Self Calculation 5/APF & Reference Correction ==
  Reference : Inport
  Obstacle Information : Inport  Port=2
  Position : Inport  Port=3
  Velocity : Inport  Port=4
  Constant : Constant  Value=0
  Constant1 : Constant  Value=[0;0]
  Find closest obstacle : MATLAB Function  TreatAsAtomicUnit=on
  Manual Switch : ManualSwitch  CurrentSetting=0
  Manual Switch1 : ManualSwitch
  Scope : Scope
  Scope1 : Scope
  Subsystem : Subsystem
  f_ik : Outport
  delta_x : Outport  Port=2
  delta_v : Outport  Port=3
  ddot_x_d : Outport  Port=4
  wires:
  Position/1 -> Subsystem/3(Position), Find closest obstacle/2(pos)
  Obstacle Information/1 -> Subsystem/2(Obstacle Information), Find closest obstacle/1(ob_info)
  Find closest obstacle/1(flag_ob) -> Manual Switch/2
  Constant/1 -> Manual Switch/1
  Manual Switch/1 -> Scope1/1, Subsystem/5(Flag_ob)
  Reference/1 -> Subsystem/1(Reference)
  Subsystem/3(ddot_x_d) -> ddot_x_d/1
  Subsystem/2(delta_v) -> delta_v/1
  Subsystem/1(delta_x) -> delta_x/1
  Velocity/1 -> Subsystem/4(Velocity)
  Find closest obstacle/2(f_ik) -> Manual Switch1/1
  Constant1/1 -> Manual Switch1/2
  Manual Switch1/1 -> Scope/1, f_ik/1

== system five_bots_Observer_Obstacle_1_sin_cir/Self Calculation 5/Observation and selection ==
  u : Inport
  Velocity : Inport  Port=2
  Position : Inport  Port=3
  Control input transfer : MATLAB Function  TreatAsAtomicUnit=on
  Observer : Subsystem
  Scope2 : Scope
  Selecting Information : MATLAB Function  TreatAsAtomicUnit=on
  Ob_estimation : Outport
  d_hat : Outport  Port=2
  wires:
  Selecting Information/1(ob_estimation) -> Ob_estimation/1
  Observer/2(second_hat) -> Selecting Information/2(second_hat)
  Observer/1(first_hat) -> Selecting Information/1(first_hat)
  Observer/3(first_hat_dot) -> Selecting Information/3(first_hat_dot)
  Position/1 -> Control input transfer/2(pos), Observer/3(Position)
  Velocity/1 -> Observer/2(Velocity)
  Control input transfer/1(u_norm) -> Scope2/1, Observer/1(u_norm)
  u/1 -> Control input transfer/1(u)
  Selecting Information/2(d_hat) -> d_hat/1

== system five_bots_Observer_Obstacle_1_sin_cir/Self Calculation 1/APF & Reference Correction/Subsystem ==
  Reference : Inport
  Obstacle Information : Inport  Port=2
  Position : Inport  Port=3
  Velocity : Inport  Port=4
  Flag_ob : Inport  Port=5
  Abstract : MATLAB Function  TreatAsAtomicUnit=on
  Error calculation : MATLAB Function  TreatAsAtomicUnit=on
  Reference Correction : MATLAB Function  TreatAsAtomicUnit=on
  Scope : Scope
  Scope1 : Scope
  delta_x : Outport
  delta_v : Outport  Port=2
  ddot_x_d : Outport  Port=3
  wires:
  Reference/1 -> Abstract/1(reference)
  Error calculation/1(delta_x) -> delta_x/1
  Error calculation/2(delta_v) -> delta_v/1
  Abstract/1(agent_x_d) -> Reference Correction/1(agent_x_d)
  Abstract/2(agent_dot_x_d) -> Reference Correction/2(agent_dot_x_d)
  Abstract/3(agent_ddot_x_d) -> Reference Correction/3(agent_ddot_x_d)
  Obstacle Information/1 -> Reference Correction/4(ob_info)
  Position/1 -> Error calculation/3(pos), Reference Correction/5(pos)
  Velocity/1 -> Error calculation/4(vel), Reference Correction/6(vel)
  Flag_ob/1 -> Reference Correction/7(flag_ob)
  Reference Correction/1(new_x_d) -> Scope/1, Error calculation/1(agent_x_d)
  Reference Correction/2(new_dot_x_d) -> Error calculation/2(agent_dot_x_d)
  Reference Correction/3(new_ddot_x_d) -> ddot_x_d/1
  Reference Correction/4(k_i) -> Scope1/1

== system five_bots_Observer_Obstacle_1_sin_cir/Self Calculation 1/Observation and selection/Observer ==
  u_norm : Inport
  Velocity : Inport  Port=2
  Position : Inport  Port=3
  Integrator : Integrator  InitialCondition=[-0;0.8;pi/6;0;0;0;0;0;0]  ContinuousStateAttributes='speed'
  Integrator1 : Integrator  InitialCondition=[0;0;0;0;0;0;0;0;0]  ContinuousStateAttributes='speed'
  Memory : Memory  InitialCondition=[0;0;0;0;0;0;0;0;0]  LinearizeMemory=on
  Observer : MATLAB Function  TreatAsAtomicUnit=on
  first_hat : Outport
  second_hat : Outport  Port=2
  first_hat_dot : Outport  Port=3
  wires:
  Velocity/1 -> Observer/2(vel)
  Integrator/1 -> first_hat/1, Observer/4(first_hat)
  u_norm/1 -> Observer/3(u_norm)
  Observer/1(first_hat_dot) -> Memory/1, Integrator/1
  Position/1 -> Observer/1(pos)
  Observer/2(second_hat_dot) -> Integrator1/1
  Integrator1/1 -> second_hat/1, Observer/5(second_hat)
  Memory/1 -> first_hat_dot/1

== system five_bots_Observer_Obstacle_1_sin_cir/Self Calculation 2/APF & Reference Correction/Subsystem ==
  Reference : Inport
  Obstacle Information : Inport  Port=2
  Position : Inport  Port=3
  Velocity : Inport  Port=4
  Flag_ob : Inport  Port=5
  Abstract : MATLAB Function  TreatAsAtomicUnit=on
  Error calculation : MATLAB Function  TreatAsAtomicUnit=on
  Reference Correction : MATLAB Function  TreatAsAtomicUnit=on
  Scope : Scope
  Scope1 : Scope
  delta_x : Outport
  delta_v : Outport  Port=2
  ddot_x_d : Outport  Port=3
  wires:
  Reference/1 -> Abstract/1(reference)
  Error calculation/1(delta_x) -> delta_x/1
  Error calculation/2(delta_v) -> delta_v/1
  Abstract/1(agent_x_d) -> Reference Correction/1(agent_x_d)
  Abstract/2(agent_dot_x_d) -> Reference Correction/2(agent_dot_x_d)
  Abstract/3(agent_ddot_x_d) -> Reference Correction/3(agent_ddot_x_d)
  Obstacle Information/1 -> Reference Correction/4(ob_info)
  Position/1 -> Error calculation/3(pos), Reference Correction/5(pos)
  Velocity/1 -> Error calculation/4(vel), Reference Correction/6(vel)
  Flag_ob/1 -> Reference Correction/7(flag_ob)
  Reference Correction/1(new_x_d) -> Error calculation/1(agent_x_d), Scope/1
  Reference Correction/2(new_dot_x_d) -> Error calculation/2(agent_dot_x_d)
  Reference Correction/3(new_ddot_x_d) -> ddot_x_d/1
  Reference Correction/4(k_i) -> Scope1/1

== system five_bots_Observer_Obstacle_1_sin_cir/Self Calculation 2/Observation and selection/Observer ==
  u_norm : Inport
  Velocity : Inport  Port=2
  Position : Inport  Port=3
  Integrator : Integrator  InitialCondition=[-1.3;1.4;pi/3;0;0;0;0;0;0]  ContinuousStateAttributes='speed'
  Integrator1 : Integrator  InitialCondition=[0;0;0;0;0;0;0;0;0]  ContinuousStateAttributes='speed'
  Memory : Memory  InitialCondition=[0;0;0;0;0;0;0;0;0]  LinearizeMemory=on
  Observer : MATLAB Function  TreatAsAtomicUnit=on
  first_hat : Outport
  second_hat : Outport  Port=2
  first_hat_dot : Outport  Port=3
  wires:
  Velocity/1 -> Observer/2(vel)
  Integrator/1 -> first_hat/1, Observer/4(first_hat)
  u_norm/1 -> Observer/3(u_norm)
  Observer/1(first_hat_dot) -> Memory/1, Integrator/1
  Position/1 -> Observer/1(pos)
  Observer/2(second_hat_dot) -> Integrator1/1
  Integrator1/1 -> second_hat/1, Observer/5(second_hat)
  Memory/1 -> first_hat_dot/1

== system five_bots_Observer_Obstacle_1_sin_cir/Self Calculation 3/APF & Reference Correction/Subsystem ==
  Reference : Inport
  Obstacle Information : Inport  Port=2
  Position : Inport  Port=3
  Velocity : Inport  Port=4
  Flag_ob : Inport  Port=5
  Abstract : MATLAB Function  TreatAsAtomicUnit=on
  Error calculation : MATLAB Function  TreatAsAtomicUnit=on
  Reference Correction : MATLAB Function  TreatAsAtomicUnit=on
  Scope : Scope
  Scope1 : Scope
  delta_x : Outport
  delta_v : Outport  Port=2
  ddot_x_d : Outport  Port=3
  wires:
  Reference/1 -> Abstract/1(reference)
  Error calculation/1(delta_x) -> delta_x/1
  Error calculation/2(delta_v) -> delta_v/1
  Abstract/1(agent_x_d) -> Reference Correction/1(agent_x_d)
  Abstract/2(agent_dot_x_d) -> Reference Correction/2(agent_dot_x_d)
  Abstract/3(agent_ddot_x_d) -> Reference Correction/3(agent_ddot_x_d)
  Obstacle Information/1 -> Reference Correction/4(ob_info)
  Position/1 -> Error calculation/3(pos), Reference Correction/5(pos)
  Velocity/1 -> Error calculation/4(vel), Reference Correction/6(vel)
  Flag_ob/1 -> Reference Correction/7(flag_ob)
  Reference Correction/1(new_x_d) -> Error calculation/1(agent_x_d), Scope/1
  Reference Correction/2(new_dot_x_d) -> Error calculation/2(agent_dot_x_d)
  Reference Correction/3(new_ddot_x_d) -> ddot_x_d/1
  Reference Correction/4(k_i) -> Scope1/1

== system five_bots_Observer_Obstacle_1_sin_cir/Self Calculation 3/Observation and selection/Observer ==
  u_norm : Inport
  Velocity : Inport  Port=2
  Position : Inport  Port=3
  Integrator : Integrator  InitialCondition=[-1.4;-1.2;-pi/4;0;0;0;0;0;0]  ContinuousStateAttributes='speed'
  Integrator1 : Integrator  InitialCondition=[0;0;0;0;0;0;0;0;0]  ContinuousStateAttributes='speed'
  Memory : Memory  InitialCondition=[0;0;0;0;0;0;0;0;0]  LinearizeMemory=on
  Observer : MATLAB Function  TreatAsAtomicUnit=on
  first_hat : Outport
  second_hat : Outport  Port=2
  first_hat_dot : Outport  Port=3
  wires:
  Velocity/1 -> Observer/2(vel)
  Integrator/1 -> first_hat/1, Observer/4(first_hat)
  u_norm/1 -> Observer/3(u_norm)
  Observer/1(first_hat_dot) -> Memory/1, Integrator/1
  Position/1 -> Observer/1(pos)
  Observer/2(second_hat_dot) -> Integrator1/1
  Integrator1/1 -> second_hat/1, Observer/5(second_hat)
  Memory/1 -> first_hat_dot/1

== system five_bots_Observer_Obstacle_1_sin_cir/Self Calculation 4/APF & Reference Correction/Subsystem ==
  Reference : Inport
  Obstacle Information : Inport  Port=2
  Position : Inport  Port=3
  Velocity : Inport  Port=4
  Flag_ob : Inport  Port=5
  Abstract : MATLAB Function  TreatAsAtomicUnit=on
  Error calculation : MATLAB Function  TreatAsAtomicUnit=on
  Reference Correction : MATLAB Function  TreatAsAtomicUnit=on
  Scope : Scope
  Scope1 : Scope
  delta_x : Outport
  delta_v : Outport  Port=2
  ddot_x_d : Outport  Port=3
  wires:
  Reference/1 -> Abstract/1(reference)
  Error calculation/1(delta_x) -> delta_x/1
  Error calculation/2(delta_v) -> delta_v/1
  Abstract/1(agent_x_d) -> Reference Correction/1(agent_x_d)
  Abstract/2(agent_dot_x_d) -> Reference Correction/2(agent_dot_x_d)
  Abstract/3(agent_ddot_x_d) -> Reference Correction/3(agent_ddot_x_d)
  Obstacle Information/1 -> Reference Correction/4(ob_info)
  Position/1 -> Error calculation/3(pos), Reference Correction/5(pos)
  Velocity/1 -> Error calculation/4(vel), Reference Correction/6(vel)
  Flag_ob/1 -> Reference Correction/7(flag_ob)
  Reference Correction/1(new_x_d) -> Error calculation/1(agent_x_d), Scope/1
  Reference Correction/2(new_dot_x_d) -> Error calculation/2(agent_dot_x_d)
  Reference Correction/3(new_ddot_x_d) -> ddot_x_d/1
  Reference Correction/4(k_i) -> Scope1/1
